simulink model "fig2_50_simulink"  (R2021b)
settings: Solver=ode45  StartTime=0.0  StopTime=20  RelTol=1e-3  EnableMultiTasking=on
settings Model: Creator=One Informatic  LastModifiedBy=One Informatic
settings DataIOCC: LimitDataPoints=on  SaveFormat=Array  SignalLoggingSaveFormat=ModelDataLogs  ReturnWorkspaceOutputs=off  SignalLoggingName=sigsOut
settings DebuggingCC: SaveWithParameterizedLinksMsg=none  UnderspecifiedInitializationDetection=Classic  MergeDetectMultiDrivingBlocksExec=none  SignalResolutionControl=TryResolveAllWithWarning  MultiTaskDSMMsg=warning  MultiTaskCondExecSysMsg=none
settings HardwareCC: ProdBitPerPointer=32  ProdBitPerSizeT=32  ProdBitPerPtrDiffT=32  ProdLargestAtomicFloat=None  ProdIntDivRoundTo=Undefined  ProdEndianess=Unspecified  ProdWordSize=32  ProdHWDeviceType=32-bit Generic  TargetUnknown=on
settings ModelReferenceCC: PropagateSignalLabelsOutOfModel=off
settings GRTTargetCC: CombineOutputUpdateFcns=off  GRTInterface=on
settings ConfigComp: CovMetricSettings=dw  CovSaveCumulativeToWorkspaceVar=on  CovSaveSingleToWorkspaceVar=on

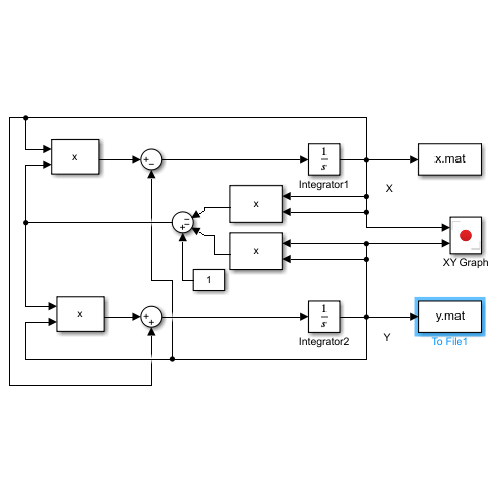
[thumbnail: Simulink's stored preview of the top-level diagram]
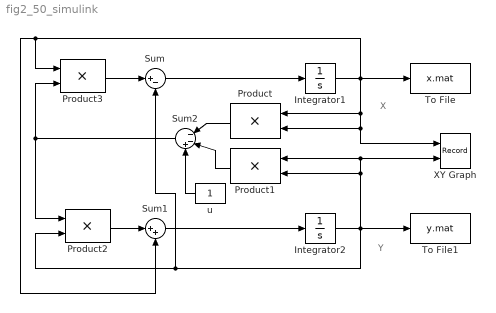
== system fig2_50_simulink ==
  note: X
  note: Y
  Integrator1 : Integrator  InitialCondition=1.8
  Integrator2 : Integrator  InitialCondition=1.8
  Product{,1..3} (4 alike) : Product  SaturateOnIntegerOverflow=on  OutDataTypeStr=Inherit: Same as first input
  Sum : Sum  Inputs=|+-  SaturateOnIntegerOverflow=on
  Sum1 : Sum  Inputs=|++  SaturateOnIntegerOverflow=on
  Sum2 : Sum  Inputs=|--+  SaturateOnIntegerOverflow=on
  To File : ToFile  Filename=x.mat  MatrixName=x  SampleTime=0.001
  To File1 : ToFile  Filename=y.mat  MatrixName=y  SampleTime=0.001
  XY Graph : Record  FileSettingsInternal="{\"entries\":[{\"content\":{\"excelSettings\":{\"content\":{},\"type\":\"Streamout.ExcelSettings\"}},\"type\":\"Streamout.FileSettingStorage\",\"uuid\":\"dae918f3-7d2f-479d-a086-fab08fd9a2cf\"}],\"packageUris\":[\"http://schema.mathworks.com/mf0/streamout_blocks/R2020a\"],\"version\":\"1.0\"}"  Layout=[1 1]  SignalsInternal="{\"entries\":[{\"content\":{\"signals\":[{\"content\":{\"blockPath\":[\"fig2_50_simulink/XY Graph\"],\"channel\":[],\"dimensions\":[1],\"domain\":\"fig2_50_simulink/XY Graph\",\"lineColor\":\"#0072bd\",\"plots\":[],\"port\":1,\"sid\":[\"\"],\"signalID\":105,\"signalName\":\"Integrator1\"},\"type\":\"RecordBlkView.Signal\",\"uuid\":\"44b29ade-b787-4e18-b852-6404ba3b93e4\"},{\"content\":{\"blockPath\":[\"fig2_50_simulink/XY Graph\"],\"channel\":[],\"dimensions\":[1],\"domain\":\"fig2_50_simulink/XY Graph\",\"lineColor\":\"#d95319\",\"plots\":[],\"port\":2,\"sid\":[\"\"],\"signalID\":109,\"signalName\":\"Integrator2\"},\"type\":\"RecordBlkView.Signal\",\"uuid\":\"17962c39-497f-48ac-98ca-9969d9ce09b1\"}]},\"type\":\"RecordBlkView.InputSignals\",\"uuid\":\"f017c0e5-75bb-4054-8688-95e4a5199e4a\"}],\"packageUris\":[\"http://schema.mathworks.com/mf0/streamout_blocks/R2020a\"],\"version\":\"1.0\"}"  VisualizationBindings="{\"xyplotplugin\":{\"info\":[{\"series\":[],\"subplotID\":1}]}}"  CompatibilityTag=XY  st=0.02
  u : Constant
  wires:
  Product/1 -> Sum2/1
  Product1/1 -> Sum2/2
  u/1 -> Sum2/3
  Integrator1/1 -> To File/1, Product/1, Product/2, XY Graph/1, Product3/1, Sum1/2
  Sum2/1 -> Product3/2, Product2/1
  Sum/1 -> Integrator1/1
  Product3/1 -> Sum/1
  Sum1/1 -> Integrator2/1
  Product2/1 -> Sum1/1
  Integrator2/1 -> To File1/1, Product1/1, XY Graph/2, Product1/2, Product2/2, Sum/2
